simulink library "S_TaLiRo"  (R2013b)
settings: Solver=ode45  StartTime=0.0  StopTime=10.0  RelTol=1e-3
undefined symbols (not defined in the file): phi_for_sfunction_use_only, pred_for_sfunction_use_only
settings Model: Creator=adokhanc  LastModifiedBy=adokhanc

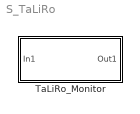
== system S_TaLiRo ==
  TaLiRo_Monitor : Subsystem  StopFcn=|  mask(Parameters){sample=1, specnm=Phi, predmp=Pred}
      | clear phi_for_sfunction_use_only;
      | clear pred_for_sfunction_use_only;
      mask prompts: sample "SampleTime"; specnm "SpecificationName"; predmp "PredicateMap"
      mask help:
      | SampleTime is a real value.
      | SpecificationName is a string of the form "phi" or "phi{i}" where i is a
      | positive integer.
      | The PredicateMap is a string like "pred".
      | SpecificationName and PredicateMap must be defined in the Matlab Workspace. See help for instructions.
      mask init:
      | try
      |     evalin('base','phi_for_sfunction_use_only')
      |     errordlg('Variable phi_for_sfunction_use_only is a reserved name for internal use')
      |     stop
      | catch ME
      | end
      | try
      |     evalin('base','pred_for_sfunction_use_only')
      |     errordlg('Variable pred_for_sfunction_use_only is a reserved name for internal use')
      |     stop
      | catch ME
      | end
      | y = evalin('base',num2str(specnm));
      | assignin('base','phi_for_sfunction_use_only',y);
      | x = evalin('base',num2str(predmp));
      | assignin('base','pred_for_sfunction_use_only',x);
      mask Help: web( 'TaLiRo_help.html' )
      mask DialogControl ParameterTabVar0 Prompt: Parameters

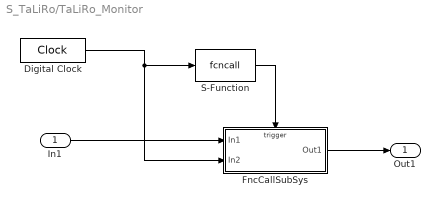
== system S_TaLiRo/TaLiRo_Monitor ==
  In1 : Inport
  Digital Clock : DigitalClock  SampleTime=sample
  FncCallSubSys : Subsystem  TreatAsAtomicUnit=on
  S-Function : S-Function  FunctionName=fcncall  Parameters=sample  EnableBusSupport=off
  Out1 : Outport
  wires:
  In1/1 -> FncCallSubSys/1(In1)
  Digital Clock/1 -> FncCallSubSys/2(In2), S-Function/1
  S-Function/1 -> FncCallSubSys/Trigger
  FncCallSubSys/1(Out1) -> Out1/1

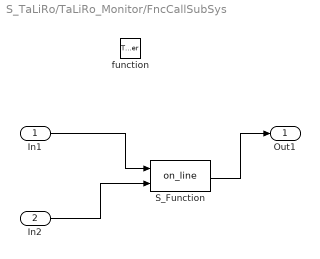
== system S_TaLiRo/TaLiRo_Monitor/FncCallSubSys ==
  In1 : Inport
  In2 : Inport  Port=2
  function : TriggerPort  TriggerType=function-call
  S_Function : S-Function  FunctionName=on_line  Parameters=phi_for_sfunction_use_only,pred_for_sfunction_use_only,sample  EnableBusSupport=off
  Out1 : Outport
  wires:
  In1/1 -> S_Function/1
  In2/1 -> S_Function/2
  S_Function/1 -> Out1/1
